simulink model "bio_matfunc_allocateThrust"  (R2017b)
settings: Solver=VariableStepAuto  StartTime=0.0  StopTime=10.0  RelTol=1e-3
settings Model: Creator=ktrinh  LastModifiedBy=ktrinh

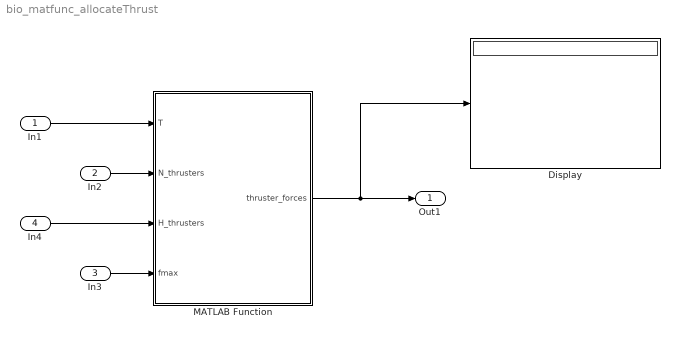
== system bio_matfunc_allocateThrust ==
  In1 : Inport  OutDataTypeStr=double  PortDimensions=3
  In2 : Inport  Port=2  OutDataTypeStr=double  PortDimensions=1
  In3 : Inport  Port=3  OutDataTypeStr=double  PortDimensions=1
  In4 : Inport  Port=4  OutDataTypeStr=double  PortDimensions=[6,6]
  Display : Display
  MATLAB Function : MATLAB Function  TreatAsAtomicUnit=on
  Out1 : Outport
  wires:
  In1/1 -> MATLAB Function/1(T)
  In2/1 -> MATLAB Function/2(N_thrusters)
  In3/1 -> MATLAB Function/4(fmax)
  In4/1 -> MATLAB Function/3(H_thrusters)
  MATLAB Function/1(thruster_forces) -> Display/1, Out1/1

== matlab function bio_matfunc_allocateThrust/MATLAB Function ==
  data: T input; N_thrusters input; thruster_forces output; H_thrusters input; fmax input
function thruster_forces = allocateThrust(T,N_thrusters,H_thrusters,fmax)
%#codegen

thruster_forces = zeros(6,1);
H = H_thrusters(4:6,:);
usat = zeros(6,1);
u = zeros(6,1);
flag = 0;
while flag == 0
    flag = 1;
    %u = pinv(H)*T;
    u = H'*inv(H*H')*T;
    for j = 1:N_thrusters
        if u(j) < -0.000000001
            u(j) = 0;
            %usat(j) = 0;
            %T = T - H*usat;
            H(:,j) = zeros(3,1);
            flag = 0;
        end
    end
end
%u = u + usat;
thruster_forces = u;
